simulink model "Fault_Tolerant_Motor_Control"  (R2023b)
settings: Solver=ode23  StartTime=0.0  StopTime=1  RelTol=1e-7
values from neighbouring files (symbols this model uses):
  a = 0.01    [Parameters.m]
  Fc_EMF = 60    [Parameters.m]
  Imax = 95    [Parameters.m]
  J = 0.01    [Parameters.m]
  K_SMO = 20    [Parameters.m]
  Kb_PLL = 50    [Parameters.m]
  Ki_PLL = 9    [Parameters.m]
  Ki_w = 210    [Parameters.m]
  Kp_PLL = 1    [Parameters.m]
  Kp_w = 2.9    [Parameters.m]
  Ld = 0.00047    [Parameters.m]
  Lq = 0.00047    [Parameters.m]
  m = 0.06    [Parameters.m]
  P = 4    [Parameters.m]
  Pmax = 50000    [Parameters.m]
  Psi = 0.1    [Parameters.m]
  Rs = 0.079    [Parameters.m]
  Te_max = 80    [Parameters.m]
  theta_offset = 0    [Parameters.m]
  Ts = 2e-6    (= 2e-06)    [Parameters.m]
  Tsc = 5e-05    [Parameters.m]
  Vdc = 370    [Parameters.m]
undefined symbols (not defined in the file or in its folder): DiscIntNeverNeededParam, ee_sli_rtmsupport, gcbh
libraries: fl_lib x18, nesl_utility x17, ee_lib x11, simulink x6, eeTransforms x2, mcbcontrolslib x2, eePmsmCurrentController x1, eePwmGeneratorTwoLevel x1, slpidlib x1, eeDiscretePi x1, batteryecm_lib x1, eeResolverToDigitalConverter x1
(part 2 of 2)

== system Fault_Tolerant_Motor_Control/Controller/Measurment Scope/Position Error ==
  Add : Sum  Inputs=+-
  Out1 : Outport
  wires:
  Add/1 -> Out1/1
  [theta_e_est_PLL] -> Add/2  "Estimated Electrical Position (rad)"
  [theta_e] -> Add/1  "Resolver Electrical Angle (rad)"

== system Fault_Tolerant_Motor_Control/Controller/Measurment Scope/Speed Error ==
  Add : Sum  Inputs=+-
  Out1 : Outport
  wires:
  Add/1 -> Out1/1
  [Wm_est_PLL] -> Add/2  "Estimated Mechanical Speed (rad/s)"
  [Wm] -> Add/1  "Resolver Mechanical Speed (rad/s)"

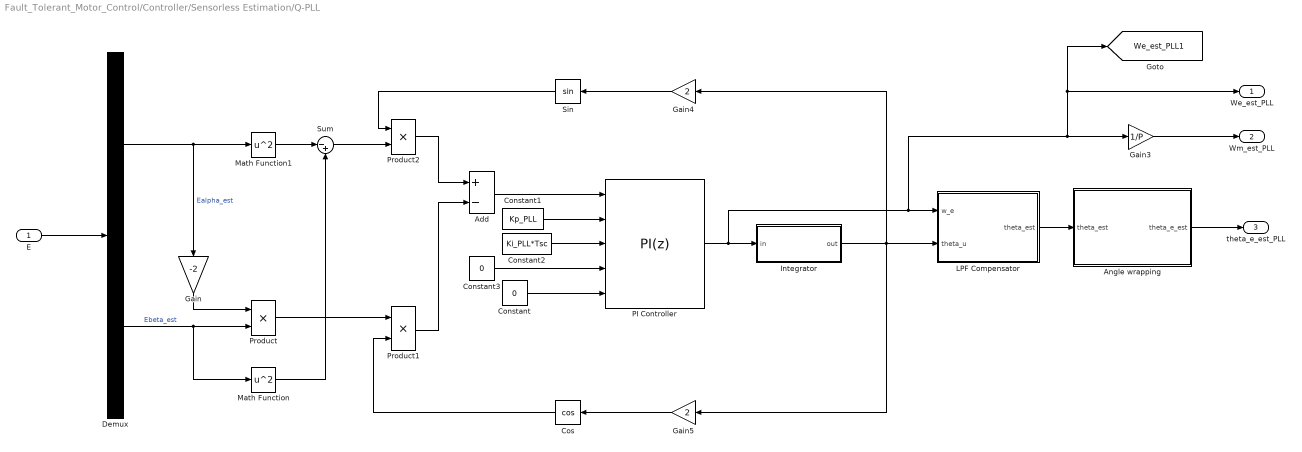
== system Fault_Tolerant_Motor_Control/Controller/Sensorless Estimation/Q-PLL ==
  E : Inport
  Add : Sum  Inputs=+-
  Angle wrapping : Subsystem
  Constant : Constant  Value=0
  Constant1 : Constant  Value=Kp_PLL
  Constant2 : Constant  Value=Ki_PLL*Tsc
  Constant3 : Constant  Value=0
  Cos : Trigonometry  Operator=cos
  Demux : Demux  Outputs=2
  Gain : Gain  Gain=-2
  Gain3 : Gain  Gain=1/P
  Gain4 : Gain  Gain=2
  Gain5 : Gain  Gain=2
  Integrator : Subsystem
  LPF Compensator : Subsystem
  Math Function : Math  Operator=square
  Math Function1 : Math  Operator=square
  PI Controller : slpidlib/PID Controller  Controller=PI  Form=Parallel  TimeDomain=Discrete-time  UseExternalTs=off  SampleTime=-1  IntegratorMethod=Forward Euler  FilterMethod=Forward Euler  ControllerParametersSource=external  P=1  I=1  UseKiTs=on  D=0  N=100  UseFilter=on  TunerSelectOption=Transfer Function Based (PID Tuner App)  InitialConditionSource=external  InitialConditionForIntegrator=0  InitialConditionForFilter=0  DifferentiatorICPrevScaledInput=0  ExternalReset=level  TrackingMode=off  Kt=1  LimitOutput=on  SatLimitsSource=internal  UpperSaturationLimit=3000  LowerSaturationLimit=-3000  LinearizeAsGain=on  AntiWindupMode=back-calculation  Kb=Kb_PLL  LimitIntegrator=off  UpperIntegratorSaturationLimit=inf  LowerIntegratorSaturationLimit=-inf  POutMin=[]  POutMax=[]  IOutMin=[]  IOutMax=[]  DOutMin=[]  DOutMax=[]  NOutMin=[]  NOutMax=[]  SumOutMin=[]  SumOutMax=[]  SaturationOutMin=[]  SaturationOutMax=[]  PParamMin=[]  PParamMax=[]  IParamMin=[]  IParamMax=[]  DParamMin=[]  DParamMax=[]  NParamMin=[]  NParamMax=[]  KbParamMin=[]  KbParamMax=[]  KtParamMin=[]  KtParamMax=[]  KbOutMin=[]  KbOutMax=[]  KtOutMin=[]  KtOutMax=[]  IntegratorOutMin=[]  IntegratorOutMax=[]  FilterOutMin=[]  FilterOutMax=[]  SumI1OutMin=[]  SumI1OutMax=[]  SumI2OutMin=[]  SumI2OutMax=[]  SumI3OutMin=[]  SumI3OutMax=[]  SumI4OutMin=[]  SumI4OutMax=[]  SumDOutMin=[]  SumDOutMax=[]  DifferentiatorOutMin=[]  DifferentiatorOutMax=[]  FilterDiffOutCoefMin=[]  FilterDiffOutCoefMax=[]  ReciprocalOutMin=[]  ReciprocalOutMax=[]  SumDenOutMin=[]  SumDenOutMax=[]  SumNumOutMin=[]  SumNumOutMax=[]  DivideOutMin=[]  DivideOutMax=[]  UdiffTsProdOutMin=[]  UdiffTsProdOutMax=[]  NTsProdOutMin=[]  NTsProdOutMax=[]  UintegralTsProdOutMin=[]  UintegralTsProdOutMax=[]  UngainTsProdOutMin=[]  UngainTsProdOutMax=[]  ClampingZeroOutDataTypeStr=Inherit: Inherit via back propagation  ClampingZeroOutMin=[]  ClampingZeroOutMax=[]  FilterDenConstantOutDataTypeStr=Inherit: Inherit via back propagation  FilterDenConstantOutMin=[]  FilterDenConstantOutMax=[]  PCopyOutDataTypeStr=Inherit: Inherit via back propagation  PCopyOutMin=[]  PCopyOutMax=[]  NCopyOutDataTypeStr=Inherit: Inherit via back propagation  NCopyOutMin=[]  NCopyOutMax=[]  IntegratorContinuousStateAttributes=''  IntegratorStateMustResolveToSignalObject=off  IntegratorRTWStateStorageClass=Auto  FilterContinuousStateAttributes=''  FilterStateMustResolveToSignalObject=off  FilterRTWStateStorageClass=Auto  ParallelPVariant=ExternalParameters  IdealPVariant=Disabled  IVariant=ExternalParameters  DVariant=Disabled  IntegratorVariant=Discrete  SatVariant=Enabled  AWVariant=BackCalculation  PCopyVariant=Disabled  TRVariant=Disabled  FdbkBlocksVariant=Forward  IdealPFdbkVariant=Disabled  SatFdbkVariant=Disabled  DerivativeFilterVariant=Disabled  NVariant=Disabled  NCopyVariant=Disabled_SignalSpec  FilterICVariant=Disabled  IntegratorICVariant=ExternalICs  ExternalResetVariant=ExternalReset  TRSumVariant=Passthrough  SumFdbkVariant=Disabled  SumVariant=Sum_PI  TsampFilterVariant=InternalTs  TsampNgainVariant=Passthrough  TsampIntegralVariant=Disabled_SignalSpec  ExternalSaturationOutDataTypeStr=Inherit: Same as second input
  Product : Product
  Product1 : Product
  Product2 : Product
  Sin : Trigonometry
  Sum : Sum  Inputs=|-+
  We_est_PLL : Outport
  Wm_est_PLL : Outport  Port=2
  theta_e_est_PLL : Outport  Port=3
  tag scope: We_est_PLL1=global
  wires:
  E/1 -> Demux/1
  Gain/1 -> Product/1
  Demux/2 -> Math Function/1, Product/2  "Ebeta_est"
  Product/1 -> Product1/1
  Demux/1 -> Gain/1, Math Function1/1  "Ealpha_est"
  Math Function1/1 -> Sum/1
  Math Function/1 -> Sum/2
  Product1/1 -> Add/2
  Sum/1 -> Product2/2
  Product2/1 -> Add/1
  Sin/1 -> Product2/1
  Cos/1 -> Product1/2
  Constant/1 -> PI Controller/5
  PI Controller/1 -> Integrator/1(in), LPF Compensator/1(w_e), Gain3/1, We_est_PLL/1, [We_est_PLL1]
  Constant1/1 -> PI Controller/2
  Constant2/1 -> PI Controller/3
  Constant3/1 -> PI Controller/4
  LPF Compensator/1(theta_est) -> Angle wrapping/1(theta_est)
  Angle wrapping/1(theta_e_est) -> theta_e_est_PLL/1
  Integrator/1(out) -> Gain4/1, LPF Compensator/2(theta_u), Gain5/1
  Gain4/1 -> Sin/1
  Gain5/1 -> Cos/1
  Add/1 -> PI Controller/1
  Gain3/1 -> Wm_est_PLL/1

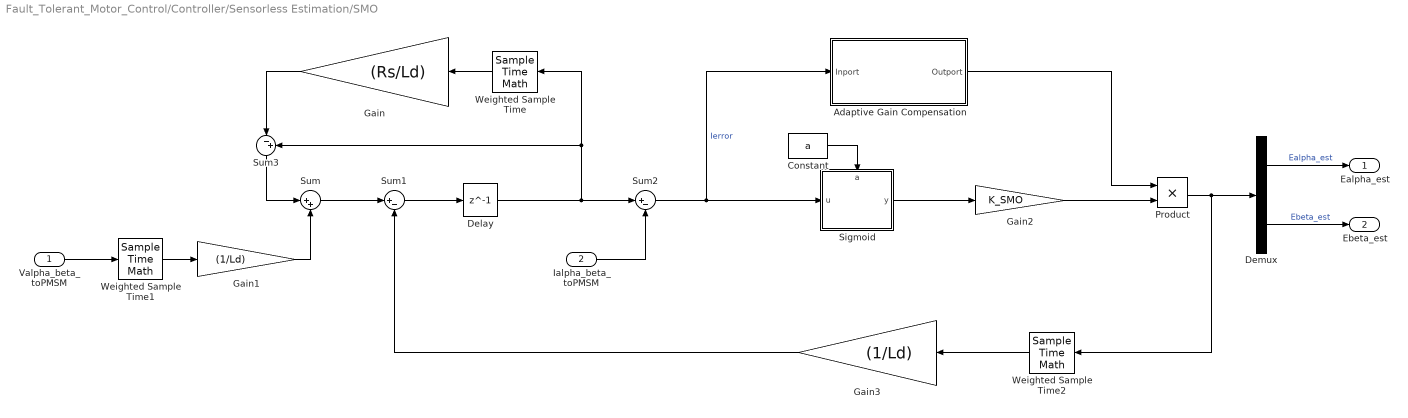
== system Fault_Tolerant_Motor_Control/Controller/Sensorless Estimation/SMO ==
  Valpha_beta_toPMSM : Inport
  Ialpha_beta_toPMSM : Inport  Port=2
  Adaptive Gain Compensation : Subsystem
  Constant : Constant  Value=a
  Delay : Delay  DelayLength=1
  Demux : Demux  Outputs=2
  Gain : Gain  Gain=(Rs/Ld)
  Gain1 : Gain  Gain=(1/Ld)
  Gain2 : Gain  Gain=K_SMO
  Gain3 : Gain  Gain=(1/Ld)
  Product : Product
  Sigmoid : Subsystem
      settings: PortSchema="{\"entries\":[{\"content\":{\"sides\":[{\"content\":{\"connectorIds\":[\"In1\"]},\"type\":\"ConnectorPlacement.EquallySpacedRectSide\",\"uuid\":\"4184fe01-1c54-4a58-b578-546864c1fbde\"},{\"content\":{\"connectorIds\":[\"Out1\"],\"side\":\"RIGHT\"},\"type\":\"ConnectorPlacement.EquallySpacedRectSide\",\"uuid\":\"8bbd5052-c9e2-4bbb-a921-3dcf5babc961\"},{\"content\":{\"connectorIds\":[\"In2\"],\"side\":\"TOP\"},\"type\":\"ConnectorPlacement.EquallySpacedRectSide\",\"uuid\":\"8f0e33aa-52cf-49ef-bc7c-6f87b0596942\"}]},\"type\":\"ConnectorPlacement.EquallySpacedConnector\",\"uuid\":\"89ccffba-4b3a-4cea-b8ab-91c287d974d8\"}],\"packageUris\":[\"http://schema.mathworks.com/mf0/Connector/R2020b\"],\"version\":\"1.0\"}"
  Sum : Sum  Inputs=|++
  Sum1 : Sum  Inputs=|+-
  Sum2 : Sum  Inputs=|+-
  Sum3 : Sum  Inputs=|-+
  Weighted Sample Time : SampleTimeMath  TsampMathOp=*
  Weighted Sample Time1 : SampleTimeMath  TsampMathOp=*
  Weighted Sample Time2 : SampleTimeMath  TsampMathOp=*
  Ealpha_est : Outport
  Ebeta_est : Outport  Port=2
  wires:
  Constant/1 -> Sigmoid/2(a)
  Product/1 -> Weighted Sample Time2/1, Demux/1
  Gain3/1 -> Sum1/2
  Gain1/1 -> Sum/2
  Gain2/1 -> Product/2
  Delay/1 -> Sum2/1, Weighted Sample Time/1, Sum3/2
  Demux/1 -> Ealpha_est/1  "Ealpha_est"
  Sigmoid/1(y) -> Gain2/1
  Weighted Sample Time/1 -> Gain/1
  Weighted Sample Time2/1 -> Gain3/1
  Valpha_beta_toPMSM/1 -> Weighted Sample Time1/1
  Demux/2 -> Ebeta_est/1  "Ebeta_est"
  Sum2/1 -> Adaptive Gain Compensation/1(Inport), Sigmoid/1(u)  "Ierror"
  Gain/1 -> Sum3/1
  Weighted Sample Time1/1 -> Gain1/1
  Ialpha_beta_toPMSM/1 -> Sum2/2
  Sum/1 -> Sum1/1
  Sum3/1 -> Sum/1
  Sum1/1 -> Delay/1
  Adaptive Gain Compensation/1(Outport) -> Product/1

== system Fault_Tolerant_Motor_Control/Controller/Sensorless Estimation/Second Order LPF ==
  x : Inport
  Compute a : Subsystem
  Demux : Demux  Outputs=2
  Scope : Scope  NumInputPorts=2
  Subsystem : Subsystem
  Subsystem1 : Subsystem
  y : Outport
  wires:
  x/1 -> Subsystem/1(x)
  Compute a/1(a) -> Subsystem/2(a), Subsystem1/2(a)
  Subsystem/1(y) -> Subsystem1/1(x)
  Subsystem1/1(y) -> Demux/1, y/1
  Demux/1 -> Scope/1  "Ealpha_est"
  Demux/2 -> Scope/2  "Ebeta_est"

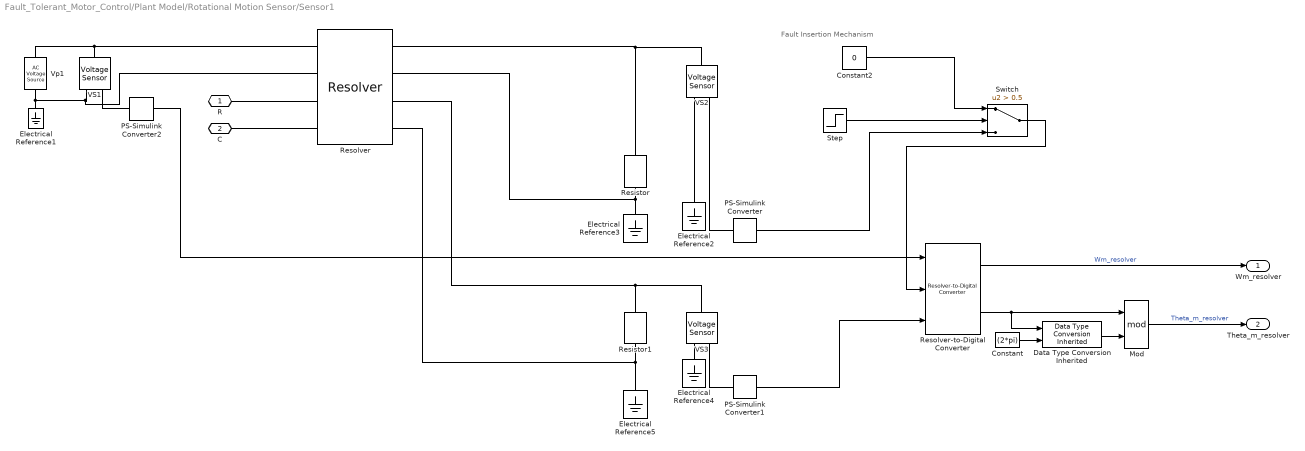
== system Fault_Tolerant_Motor_Control/Plant Model/Rotational Motion Sensor/Sensor1 ==
  note: Fault Insertion Mechanism
  Constant : Constant  Value=(2*pi)
  Constant2 : Constant  Value=0
  Data Type Conversion Inherited : simulink/Signal Attributes/Data Type Conversion Inherited  ConvertRealWorld=Real World Value  DoSatur=off
  Electrical Reference{1..5} (5 alike) : fl_lib/Electrical/Electrical Elements/Electrical Reference
  Mod : Math  Operator=mod
  PS-Simulink Converter : nesl_utility/PS-Simulink Converter  PhysicalDomain=network_engine_domain  SubClassName=ps_output  LeftPortType=input  RightPortType=output  PseudoPeriodic=off  Frequencies=[]  VectorFormat=1-D array  Unit=1  AffineConversion=off
  PS-Simulink Converter1 : nesl_utility/PS-Simulink Converter  PhysicalDomain=network_engine_domain  SubClassName=ps_output  LeftPortType=input  RightPortType=output  PseudoPeriodic=off  Frequencies=[]  VectorFormat=1-D array  Unit=1  AffineConversion=off
  PS-Simulink Converter2 : nesl_utility/PS-Simulink Converter  PhysicalDomain=network_engine_domain  SubClassName=ps_output  LeftPortType=input  RightPortType=output  PseudoPeriodic=off  Frequencies=[]  VectorFormat=1-D array  Unit=1  AffineConversion=off
  Resistor : fl_lib/Electrical/Electrical Elements/Resistor  R=1e3 Ohm  i_specify=off  i_priority=None  i=0 A  i_nominal_specify=off  i_nominal_unit=A  i_nominal_value=1  v_specify=off  v_priority=None  v=0 V  v_nominal_specify=off  v_nominal_unit=V  v_nominal_value=1
  Resistor1 : fl_lib/Electrical/Electrical Elements/Resistor  R=1e3 Ohm  i_specify=off  i_priority=None  i=0 A  i_nominal_specify=off  i_nominal_unit=A  i_nominal_value=1  v_specify=off  v_priority=None  v=0 V  v_nominal_specify=off  v_nominal_unit=V  v_nominal_value=1
  Resolver : ee_lib/Sensors & Transducers/Resolver  parameterization=1  ratio=0.5  Rr=Rs Ohm  Rs=180 Ohm  Xr=100 Ohm  Xs=300 Ohm  omega=10 kHz  Lr=0.0016 H  Ls=0.0048 H  k=0.35  N=P  theta_specify=off  theta_priority=High  theta=0 rad  theta_nominal_specify=off  theta_nominal_unit=deg  theta_nominal_value=1
      settings: InternalSimscapePortConfiguration="{\"Bottom\":[],\"Left\":[{\"id\":\"p1\",\"label\":\"p1\",\"type\":\"foundation.electrical.electrical\"},{\"id\":\"p2\",\"label\":\"p2\",\"type\":\"foundation.electrical.electrical\"},{\"id\":\"R\",\"label\":\"R\",\"type\":\"foundation.mechanical.rotational.rotational\"},{\"id\":\"C\",\"label\":\"C\",\"type\":\"foundation.mechanical.rotational.rotational\"}],\"Right\":[{\"id\":\"x1\",\"label\":\"x1\",\"type\":\"foundation.electrical.electrical\"},{\"id\":\"x2\",\"label\":\"x2\",\"type\":\"foundation.electrical.electrical\"},{\"id\":\"y1\",\"label\":\"y1\",\"type\":\"foundation.electrical.electrical\"},{\"id\":\"y2\",\"label\":\"y2\",\"type\":\"foundation.electrical.electrical\"}],\"Top\":[]}"
  Resolver-to-Digital Converter : eeResolverToDigitalConverter/Resolver-to-Digital Converter  N=P  Kp=15  Ki=2.5e5  theta0=0  Ts=Ts
  Step : Step  Time=0.7  SampleTime=0
  Switch : Switch  Criteria=u2 > Threshold  Threshold=0.5  SaturateOnIntegerOverflow=off  InputSameDT=off
  VS1 : fl_lib/Electrical/Electrical Sensors/Voltage Sensor
  VS2 : fl_lib/Electrical/Electrical Sensors/Voltage Sensor
  VS3 : fl_lib/Electrical/Electrical Sensors/Voltage Sensor
  Vp1 : fl_lib/Electrical/Electrical Sources/AC Voltage Source  amp=5 V  shift=0 rad  frequency=1e4 Hz  omega=0 rad/s
  R : PMIOPort  Side=Left
  C : PMIOPort  Port=2  Side=Left
  Wm_resolver : Outport
  Theta_m_resolver : Outport  Port=2
  wires:
  Resolver-to-Digital Converter/1 -> Wm_resolver/1  "Wm_resolver"
  Mod/1 -> Theta_m_resolver/1  "Theta_m_resolver"
  Resolver-to-Digital Converter/2 -> Data Type Conversion Inherited/1, Mod/1
  Data Type Conversion Inherited/1 -> Mod/2
  Constant/1 -> Data Type Conversion Inherited/2
  PS-Simulink Converter1/1 -> Resolver-to-Digital Converter/3
  Constant2/1 -> Switch/1
  PS-Simulink Converter2/1 -> Resolver-to-Digital Converter/1
  PS-Simulink Converter/1 -> Switch/3
  Switch/1 -> Resolver-to-Digital Converter/2
  Step/1 -> Switch/2
  connections:
  R/RConn1 -- Resolver/LConn3
  C/RConn1 -- Resolver/LConn4
  Vp1/LConn1 -- Resolver/LConn1 -- VS1/LConn1
  VS1/RConn2 -- Resolver/LConn2 -- Electrical Reference1/LConn1 -- Vp1/RConn1
  VS1/RConn1 -- PS-Simulink Converter2/LConn1
  Resistor1/LConn1 -- Resolver/RConn3 -- VS3/LConn1
  Resistor1/RConn1 -- Electrical Reference5/LConn1 -- Resolver/RConn4
  Electrical Reference3/LConn1 -- Resolver/RConn2 -- Resistor/RConn1
  Resistor/LConn1 -- Resolver/RConn1 -- VS2/LConn1
  VS3/RConn1 -- PS-Simulink Converter1/LConn1
  Electrical Reference2/LConn1 -- VS2/RConn2
  VS2/RConn1 -- PS-Simulink Converter/LConn1
  Electrical Reference4/LConn1 -- VS3/RConn2

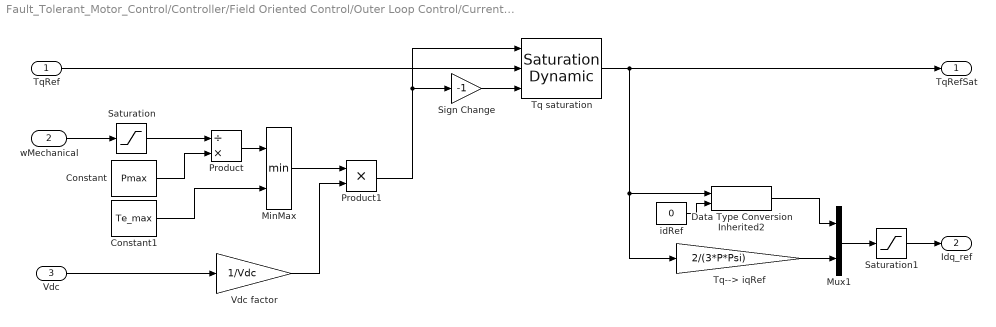
== system Fault_Tolerant_Motor_Control/Controller/Field Oriented Control/Outer Loop Control/Current Refrence Generation ==
  TqRef : Inport
  wMechanical : Inport  Port=2
  Vdc : Inport  Port=3
  Constant : Constant  Value=Pmax  SampleTime=-1
  Constant1 : Constant  Value=Te_max  SampleTime=-1
  Data Type Conversion Inherited2 : simulink/Signal Attributes/Data Type Conversion Inherited  ConvertRealWorld=Real World Value  DoSatur=off
  MinMax : MinMax  Inputs=2  OutDataTypeStr=Inherit: Same as first input
  Mux1 : Mux  Inputs=2
  Product : Product  Inputs=/*  OutDataTypeStr=Inherit: Same as first input
  Product1 : Product
  Saturation : Saturate  UpperLimit=inf  LowerLimit=(Pmax/Te_max)
  Saturation1 : Saturate  UpperLimit=Imax  LowerLimit=-Imax
  Sign Change : Gain  Gain=-1
  Tq saturation : simulink/Discontinuities/Saturation Dynamic  OutMin=[]  OutMax=[]  OutDataTypeStr=Inherit: Same as second input  OutDataType=fixdt(1, 16)  OutScaling=2^-10  DoSatur=off
  Tq--> iqRef : Gain  Gain=2/(3*P*Psi)
  Vdc factor : Gain  Gain=1/Vdc
  idRef : Constant  Value=0  SampleTime=-1
  TqRefSat : Outport  VectorParamsAs1DForOutWhenUnconnected=off
  Idq_ref : Outport  Port=2
  wires:
  Sign Change/1 -> Tq saturation/3
  Product/1 -> MinMax/1
  wMechanical/1 -> Saturation/1
  TqRef/1 -> Tq saturation/2
  Vdc factor/1 -> Product1/2
  Constant/1 -> Product/2
  Saturation/1 -> Product/1
  Vdc/1 -> Vdc factor/1
  Product1/1 -> Tq saturation/1, Sign Change/1
  MinMax/1 -> Product1/1
  Constant1/1 -> MinMax/2
  Data Type Conversion Inherited2/1 -> Mux1/1
  Tq saturation/1 -> Tq--> iqRef/1, Data Type Conversion Inherited2/1, TqRefSat/1
  Tq--> iqRef/1 -> Mux1/2
  idRef/1 -> Data Type Conversion Inherited2/2
  Mux1/1 -> Saturation1/1
  Saturation1/1 -> Idq_ref/1

== system Fault_Tolerant_Motor_Control/Controller/Field Oriented Control/Outer Loop Control/Torque Controller ==
  wRef : Inport
  wMechanical : Inport  Port=2  SampleTime=Ts
  TqRefSat : Inport  Port=3  SampleTime=Ts
  Reset : Inport  Port=4  SampleTime=Ts
  Constant7 : Constant  Value=0
  Discrete PI Controller : Subsystem  AncestorBlock=eeDiscretePi/Discrete PI Controller  LoadFcn=ee_sli_rtmsupport( 'loadfcn', gcbh );  mask(Discrete PI Controller){Kp=Kp_w, Ki=Ki_w, Kaw=800, x0=0, Ts=Tsc}
      mask prompts: Kp "physmod:ee:library:comments:control:eeDiscretePi:ProportionalGain_MP"; Ki "physmod:ee:library:comments:control:eeDiscretePi:IntegralGain_MP"; Kaw "physmod:ee:library:comments:control:eeDiscretePi:AntiwindupGain_MP"; x0 "physmod:ee:library:comments:control:eeDiscretePi:IntegratorInitialCondition_MP"; Ts "physmod:ee:library:comments:control:eeDiscretePi:SampleTime1ForInherited_MP"
      mask help: physmod:ee:library:comments:control:eeDiscretePi:DiscretePIController_MD
      mask init:
      | if Ts <= 0 && Ts ~= -1            
      |     error(message('physmod:ee:library:MinusOneOrPositive',getString(message('physmod:ee:library:comments:control:eeDiscretePi:SampleTime1ForInherited_MP'))));            
      | end
      settings: CopyFcn=ee_sli_rtmsupport( 'copyfcn', gcbh );  DeleteFcn=ee_sli_rtmsupport( 'deletefcn', gcbh );  ModelCloseFcn=ee_sli_rtmsupport( 'modelclosefcn', gcbh );  PostSaveFcn=ee_sli_rtmsupport( 'postsavefcn', gcbh );  PreCopyFcn=ee_sli_rtmsupport( 'precopyfcn', gcbh );  OpenFcn=ee_sli_rtmsupport( 'openfcn', gcbh );  CloseFcn=ee_sli_rtmsupport( 'closefcn', gcbh );  PreDeleteFcn=ee_sli_rtmsupport( 'predeletefcn', gcbh );
      mask Help: web(nesl_help(gcbh))
      mask DialogControl Container1 Prompt: physmod:ee:library:comments:control:eeDiscretePi:tab_Parameters
      mask DialogControl Kp Prompt: Proportional gain
      mask DialogControl Ki Prompt: Integral gain
      mask DialogControl Kaw Prompt: Anti-windup gain
      mask DialogControl x0 Prompt: Integrator initial condition
      mask DialogControl Ts Prompt: Sample time (-1 for inherited)
      mask Display: ee.mask.drawDiscretePi(gcb);
  Sum : Sum  Inputs=|+-
  Sum1 : Sum  Inputs=-+
  TqRefUnsat : Outport  VectorParamsAs1DForOutWhenUnconnected=off
  wires:
  TqRefSat/1 -> Sum1/2
  wMechanical/1 -> Sum/2
  Discrete PI Controller/1(u) -> TqRefUnsat/1, Sum1/1
  wRef/1 -> Sum/1
  Sum1/1 -> Discrete PI Controller/2(du)
  Reset/1 -> Discrete PI Controller/3(Reset)
  Sum/1 -> Discrete PI Controller/1(e)
  Constant7/1 -> Discrete PI Controller/4(Init0)

== system Fault_Tolerant_Motor_Control/Controller/Sensorless Estimation/Q-PLL/Angle wrapping ==
  theta_est : Inport
  Constant : Constant  Value=(2*pi)
  Data Type Conversion Inherited : simulink/Signal Attributes/Data Type Conversion Inherited  ConvertRealWorld=Real World Value  DoSatur=off
  Mod : Math  Operator=mod
  theta_e_est : Outport
  wires:
  Data Type Conversion Inherited/1 -> Mod/2
  Constant/1 -> Data Type Conversion Inherited/2
  theta_est/1 -> Data Type Conversion Inherited/1, Mod/1
  Mod/1 -> theta_e_est/1

== system Fault_Tolerant_Motor_Control/Controller/Sensorless Estimation/Q-PLL/Integrator ==
  in : Inport
  Constant : Constant  Value=(2*pi)
  Delay1 : Delay  DelayLength=1
  Delay2 : Delay  DelayLength=1
  Mod : Math  Operator=mod
  Sample time : SampleTimeMath  TsampMathOp=*
  Sum1 : Sum  Inputs=|++
  out : Outport
  wires:
  Delay1/1 -> Sum1/2
  Sample time/1 -> Sum1/1
  in/1 -> Sample time/1
  Delay2/1 -> out/1
  Sum1/1 -> Mod/1
  Mod/1 -> Delay1/1, Delay2/1
  Constant/1 -> Mod/2

== system Fault_Tolerant_Motor_Control/Controller/Sensorless Estimation/Q-PLL/LPF Compensator ==
  w_e : Inport
  theta_u : Inport  Port=2
  Add : Sum  Inputs=+++
  Atan2 : Trigonometry  Operator=atan2
  Constant : Constant  Value=(2*pi*Fc_EMF)
  Constant1 : Constant  Value=0
  Gain : Gain  Gain=2
  theta_est : Outport
  wires:
  w_e/1 -> Atan2/1
  Constant/1 -> Atan2/2
  Atan2/1 -> Gain/1
  Gain/1 -> Add/1
  theta_u/1 -> Add/2
  Add/1 -> theta_est/1
  Constant1/1 -> Add/3

== system Fault_Tolerant_Motor_Control/Controller/Sensorless Estimation/SMO/Adaptive Gain Compensation ==
  Inport : Inport
  Add : Sum
  Constant : Constant  Value=0
  Demux : Demux  Outputs=2
  Discrete PI Controller : eeDiscretePi/Discrete PI Controller  Kp=20  Ki=45  Kaw=10  x0=0  Ts=-1
      settings: LibrarySourceBlock=ee_sl_lib/General Control/Discrete PI Controller
  Gain : Gain  Gain=m
  Saturation : Saturate  UpperLimit=1200  LowerLimit=0
  Sqrt : Sqrt
  Square : Math  Operator=square
  Square1 : Math  Operator=square
  Sum : Sum  Inputs=|+-
  Sum1 : Sum  Inputs=|+-
  Outport : Outport
  wires:
  Inport/1 -> Demux/1
  Demux/1 -> Square/1  "Ialpha_err"
  Demux/2 -> Square1/1  "Ibeta_err"
  Square/1 -> Add/1
  Square1/1 -> Add/2
  Add/1 -> Sqrt/1
  Discrete PI Controller/1 -> Sum/2, Saturation/1
  Saturation/1 -> Outport/1, Gain/1, Sum/1  "Gain"
  Constant/1 -> Discrete PI Controller/3
  Sum/1 -> Discrete PI Controller/2
  Sqrt/1 -> Sum1/1
  Sum1/1 -> Discrete PI Controller/1
  Gain/1 -> Sum1/2

== system Fault_Tolerant_Motor_Control/Controller/Sensorless Estimation/SMO/Sigmoid ==
  note: (2/(1+exp(-a*u[1])))-1)
  u : Inport
  a : Inport  Port=2
  Demux : Demux  Outputs=2
  Fcn : Fcn  Expr=(2/(1+exp(-u[2]*u[1])))-1
  Fcn1 : Fcn  Expr=(2/(1+exp(-u[2]*u[1])))-1
  Mux : Mux  Inputs=2
  Mux1 : Mux  Inputs=2
  Mux2 : Mux  Inputs=2
  y : Outport
  wires:
  u/1 -> Demux/1
  Mux/1 -> y/1
  Fcn/1 -> Mux/1
  Fcn1/1 -> Mux/2
  Mux1/1 -> Fcn/1
  Demux/1 -> Mux1/1
  Demux/2 -> Mux2/1
  Mux2/1 -> Fcn1/1
  a/1 -> Mux1/2, Mux2/2

== system Fault_Tolerant_Motor_Control/Controller/Sensorless Estimation/Second Order LPF/Compute a ==
  Add : Sum  Inputs=+-
  Constant : Constant
  Constant1 : Constant
  Constant2 : Constant  Value=1 / (2*pi*Fc_EMF)
  Divide : Product  Inputs=*/
  Weighted Sample Time : SampleTimeMath  TsampMathOp=Ts Only
  Weighted Sample Time1 : SampleTimeMath  weightValue=1
  a : Outport
  wires:
  Add/1 -> a/1
  Constant/1 -> Add/1
  Constant1/1 -> Weighted Sample Time/1
  Weighted Sample Time/1 -> Divide/1
  Divide/1 -> Add/2
  Weighted Sample Time1/1 -> Divide/2
  Constant2/1 -> Weighted Sample Time1/1

== system Fault_Tolerant_Motor_Control/Controller/Sensorless Estimation/Second Order LPF/Subsystem ==
  note: y[n] = a * y[n-1] + (1-a) * x[n]
  x : Inport
  a : Inport  Port=2
  Add : Sum  Inputs=+-
  Add1 : Sum
  Delay : Delay  DelayLength=1
  Product : Product
  Product1 : Product
  y : Outport
  wires:
  x/1 -> Add/1, Product/1
  a/1 -> Product1/1, Product/2
  Product/1 -> Add/2
  Add/1 -> Add1/1
  Add1/1 -> Delay/1, y/1
  Product1/1 -> Add1/2
  Delay/1 -> Product1/2

== system Fault_Tolerant_Motor_Control/Controller/Sensorless Estimation/Second Order LPF/Subsystem1 ==
  note: y[n] = a * y[n-1] + (1-a) * x[n]
  x : Inport
  a : Inport  Port=2
  Add : Sum  Inputs=+-
  Add1 : Sum
  Delay : Delay  DelayLength=1
  Product : Product
  Product1 : Product
  y : Outport
  wires:
  x/1 -> Add/1, Product/1
  a/1 -> Product1/1, Product/2
  Product/1 -> Add/2
  Add/1 -> Add1/1
  Add1/1 -> Delay/1, y/1
  Product1/1 -> Add1/2
  Delay/1 -> Product1/2

== system Fault_Tolerant_Motor_Control/Controller/Field Oriented Control/Outer Loop Control/Torque Controller/Discrete PI Controller ==
  e : Inport  SampleTime=Ts
  du : Inport  Port=2  SampleTime=Ts
  Reset : Inport  Port=3  SampleTime=Ts
  Init0 : Inport  Port=4
  Discrete-Time Integrator : DiscreteIntegrator  IntegratorMethod=Integration: Backward Euler  ExternalReset=rising  InitialConditionSource=external  InitialCondition=x0  SampleTime=Ts  ICPrevOutput=DiscIntNeverNeededParam  ICPrevScaledInput=DiscIntNeverNeededParam
  Kaw : Gain  Gain=Kaw
  Ki : Gain  Gain=Ki
  Kp : Gain  Gain=Kp
  Sum : Sum  Inputs=|++
  Sum1 : Sum  Inputs=|++
  Unit Delay : UnitDelay  SampleTime=Ts  HasFrameUpgradeWarning=on
  u : Outport  VectorParamsAs1DForOutWhenUnconnected=off
  wires:
  Unit Delay/1 -> Kaw/1
  Reset/1 -> Discrete-Time Integrator/2
  du/1 -> Unit Delay/1
  Sum1/1 -> Discrete-Time Integrator/1
  Kaw/1 -> Sum1/2
  e/1 -> Kp/1, Ki/1
  Kp/1 -> Sum/1
  Ki/1 -> Sum1/1
  Discrete-Time Integrator/1 -> Sum/2
  Sum/1 -> u/1
  Init0/1 -> Discrete-Time Integrator/3

== stateflow chart Fault_Tolerant_Motor_Control/Controller/Fault Identification/Chart ==
  state Decrment_Count
    during:
    if count < 0
    count = 0;
    else
    count = count  - 1;
    end
  state Start
    entry:
    count = 0;
    Fault = 0;
  state Fault_Identification
    entry:
    Fault = 0;
    Wm_diff = abs(Wm - Wm_est_PLL);
    theta_e_diff = abs(theta_e_sensor - theta_e_est);
    during:
    Wm_diff = abs(Wm - Wm_est_PLL);
    theta_e_diff = abs(theta_e_sensor - theta_e_est);
  state Clear_Fault
    entry:
    Fault = 0;
    count = 0;
    during:
    Fault = 0;
    exit:
    Fault = 0;
  state Fault_Isolation
    entry:
    Fault =1;
    during:
    Fault = 1;
    Wm_diff = abs(Wm - Wm_est_PLL);
    theta_e_diff = abs(theta_e_sensor - theta_e_est)
  Start -> Fault_Identification [order 1] : [(StartSwitch == 1)&&(Fault == 0)]
  Decrment_Count -> Fault_Identification
  Fault_Identification -> Decrment_Count [order 3] : [(theta_e_diff < theta_e_diff1)&&(Wm_diff < Wm_diff1)]
  (default) -> Start
  Fault_Identification -> Fault_Identification [order 1] : [(Wm_diff > Wm_diff1)&&(theta_e_diff > theta_e_diff1)]{count = count + 1}
  Start -> Clear_Fault [order 2] : [StartSwitch == 0]
  Clear_Fault -> Start : [StartSwitch == 1]
  Fault_Identification -> Fault_Isolation [order 2] : [count >=MAX_COUNT]
  Fault_Isolation -> Clear_Fault : [StartSwitch == 0]
  data: StartSwitch input; Wm input; Wm_est_PLL input; Fault output; Wm_diff1 constant double =25; count local =0; Wm_diff local; MAX_COUNT local =10; theta_e_est input; theta_e_sensor input; theta_e_diff local; theta_e_diff1 constant double =0.7
